simulink model "sampleModel1905_3_sub_sub_sub"  (R2023a)
settings: Solver=VariableStepAuto  StartTime=0.0  StopTime=10.0  RelTol=1e-3
libraries: hdlsllib x5
settings Model: Creator=user1  LastModifiedBy=user1

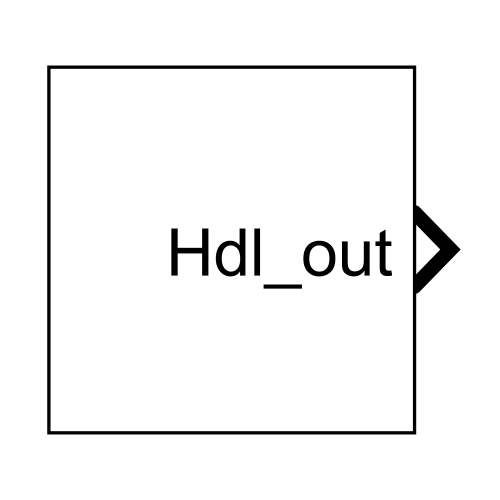
[thumbnail: Simulink's stored preview of the top-level diagram]
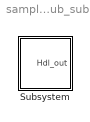
== system sampleModel1905_3_sub_sub_sub ==
  Subsystem : Subsystem

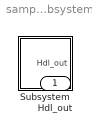
== system sampleModel1905_3_sub_sub_sub/Subsystem ==
  Subsystem : Subsystem
  Hdl_out : Outport  OutDataTypeStr=uint8

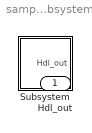
== system sampleModel1905_3_sub_sub_sub/Subsystem/Subsystem ==
  Subsystem : Subsystem
  Hdl_out : Outport  OutDataTypeStr=uint8

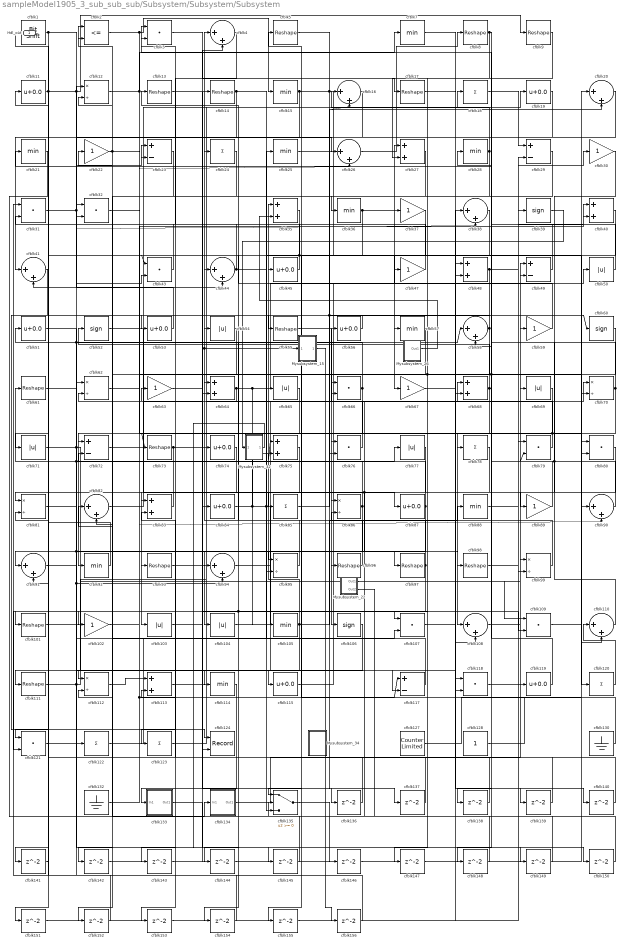
== system sampleModel1905_3_sub_sub_sub/Subsystem/Subsystem/Subsystem ==
  Mysubsystem_15 : Subsystem  TreatAsAtomicUnit=on  RTWFcnName=Mysubsystem_15
      settings: RTWFcnNameOpts=User specified  RTWFileNameOpts=Use function name
  Mysubsystem_22 : Subsystem  TreatAsAtomicUnit=on  RTWFcnName=Mysubsystem_22
      settings: RTWFcnNameOpts=User specified  RTWFileNameOpts=Use function name
  Mysubsystem_26 : Subsystem  TreatAsAtomicUnit=on  RTWFcnName=Mysubsystem_26
      settings: RTWFcnNameOpts=User specified  RTWFileNameOpts=Use function name
  Mysubsystem_32 : Subsystem  TreatAsAtomicUnit=on  RTWFcnName=Mysubsystem_32
      settings: RTWFcnNameOpts=User specified  RTWFileNameOpts=Use function name
  Mysubsystem_34 : Subsystem  TreatAsAtomicUnit=on  RTWFcnName=Mysubsystem_34
      settings: RTWFcnNameOpts=User specified  RTWFileNameOpts=Use function name
  cfblk1 : hdlsllib/Logic and Bit Operations/Bit Shift  mode=Shift Left Logical  N=0
  cfblk{5,8..9,13..14,17,55,61,73,93,96..98,101,111} (15 alike) : Reshape
  cfblk{22,30,37,47,59,63,67,89,102} (9 alike) : Gain  OutDataTypeStr=uint8
  cfblk{50,54,65,69,71,77,103..104} (8 alike) : Abs  OutDataTypeStr=uint8  SaturateOnIntegerOverflow=off
  cfblk{7,15,21,25,28,36,57,88,92,105,114} (11 alike) : MinMax  OutDataTypeStr=uint8
  cfblk{39,52,60,106} (4 alike) : Signum
  cfblk{3,31..32,43,66,76,79..80,107,109,118,121} (12 alike) : DotProduct  OutDataTypeStr=uint8
  cfblk{4,16,20,26,38,41,44,58,82,90..91,94,108,110} (14 alike) : Sum  Inputs=|++  OutDataTypeStr=uint8
  cfblk{11,19,45,51,53,56,74,84,87,115,119} (11 alike) : Bias  Bias=0.0  SaturateOnIntegerOverflow=off
  cfblk{12,62,70,81,86,95,99,112} (8 alike) : Product  Inputs=*/  OutDataTypeStr=uint8  RndMeth=Zero  SaturateOnIntegerOverflow=on
  cfblk{27,35,40,48,64,68,75,83,113} (9 alike) : Sum  OutDataTypeStr=uint8
  cfblk{23,29,49,72,117} (5 alike) : Sum  Inputs=+-  OutDataTypeStr=uint8
  cfblk{18,24,78,85,120,122..123} (7 alike) : Sum  Inputs=+  OutDataTypeStr=uint8
  cfblk124 : Record  FileSettingsInternal="{\"entries\":[{\"content\":{\"excelSettings\":{\"content\":{},\"type\":\"Streamout.ExcelSettings\"}},\"type\":\"Streamout.FileSettingStorage\",\"uuid\":\"\"}],\"packageUris\":[\"http:\\/\\/schema.mathworks.com\\/mf0\\/streamout_blocks\\/R2020a\"],\"version\":\"1.0\"}"  Layout=[1 1]  SignalsInternal="{\"entries\":[{\"content\":{\"signals\":[{\"content\":{\"blockPath\":[],\"dimensions\":[1],\"domain\":\"\",\"lineColor\":\"#a2142f\",\"plots\":[1],\"port\":1,\"signalID\":50680,\"signalName\":\"cfblk41\"},\"type\":\"RecordBlkView.Signal\",\"uuid\":\"\"},{\"content\":{\"blockPath\":[],\"dimensions\":[1],\"domain\":\"\",\"lineColor\":\"#139fff\",\"plots\":[1],\"port\":2,\"signalID\":50683,\"signalName\":\"cfblk66\"},\"type\":\"RecordBlkView.Signal\",\"uuid\":\"\"}]},\"type\":\"RecordBlkView.InputSignals\",\"uuid\":\"\"}],\"packageUris\":[\"http:\\/\\/schema.mathworks.com\\/mf0\\/streamout_blocks\\/R2020a\"],\"version\":\"1.0\"}"  VisualizationBindings="{\"xyplotplugin\":{\"info\":[{\"series\":[{\"bindingParametersList\":[{\"parameter\":\"X-Axis\",\"signalID\":50680,\"signalName\":\"cfblk41\"},{\"parameter\":\"Y-Axis\",\"signalID\":50683,\"signalName\":\"cfblk66\"}],\"seriesID\":14203}],\"subplotID\":1}]}}"  CompatibilityTag=XY  st=-1
  cfblk127 : hdlsllib/Sources/Counter Limited  uplimit=7  tsamp=-1
  cfblk128 : Constant  OutDataTypeStr=uint8  SampleTime=-1
  cfblk130 : Ground
  cfblk132 : Ground
  cfblk133 : Subsystem
      settings: LibrarySourceBlock=|
      | hdlsllib/Ports &
      | Subsystems/Subsystem
  cfblk134 : Subsystem
      settings: LibrarySourceBlock=|
      | hdlsllib/Ports &
      | Subsystems/Subsystem
  cfblk135 : Switch  OutDataTypeStr=uint8  SaturateOnIntegerOverflow=off  InputSameDT=off
  cfblk{136..156} (21 alike) : Delay  SampleTime=1
  cfblk2 : RelationalOperator  Operator=<=  OutDataTypeStr=boolean  InputSameDT=off
  Hdl_out : Outport  OutDataTypeStr=uint8
  wires:
  cfblk123/1 -> cfblk77/1
  cfblk68/1 -> cfblk152/1, cfblk28/1, cfblk52/1
  cfblk59/1 -> cfblk13/1
  cfblk96/1 -> cfblk4/1
  cfblk73/1 -> cfblk109/2, cfblk103/1
  cfblk113/1 -> cfblk19/1
  cfblk71/1 -> cfblk115/1, cfblk117/2, cfblk94/2
  cfblk102/1 -> cfblk40/1
  cfblk106/1 -> cfblk111/1
  cfblk105/1 -> cfblk114/1, cfblk88/1, cfblk35/1
  cfblk99/1 -> cfblk44/1, Mysubsystem_15/1(In1)
  cfblk2/1 -> cfblk26/2, cfblk15/1
  cfblk11/1 -> cfblk121/1, cfblk26/1, cfblk9/1
  cfblk79/1 -> cfblk73/1, cfblk5/1
  cfblk65/1 -> cfblk92/1
  cfblk26/1 -> cfblk8/1
  cfblk41/1 -> cfblk124/1
  cfblk64/1 -> cfblk62/2, cfblk105/1, cfblk50/1
  cfblk54/1 -> cfblk133/1(In1)
  cfblk115/1 -> cfblk27/1
  cfblk122/1 -> cfblk25/1
  cfblk3/1 -> cfblk17/1
  cfblk134/1(Out1) -> cfblk49/1
  cfblk21/1 -> cfblk134/1(In1)
  cfblk120/1 -> cfblk110/1
  cfblk86/1 -> cfblk155/1, cfblk65/1
  cfblk18/1 -> cfblk29/1
  cfblk57/1 -> cfblk106/1
  cfblk83/1 -> cfblk81/1
  cfblk80/1 -> cfblk86/1
  cfblk108/1 -> cfblk49/2
  cfblk93/1 -> cfblk104/1
  cfblk130/1 -> cfblk45/1
  cfblk25/1 -> cfblk120/1
  cfblk119/1 -> cfblk24/1
  cfblk30/1 -> cfblk89/1
  cfblk89/1 -> cfblk69/1
  cfblk98/1 -> cfblk39/1
  cfblk94/1 -> cfblk97/1
  cfblk109/1 -> cfblk80/1
  cfblk19/1 -> cfblk32/2
  cfblk37/1 -> cfblk55/1
  cfblk118/1 -> cfblk119/1
  cfblk52/1 -> cfblk87/1
  cfblk55/1 -> cfblk76/1
  cfblk77/1 -> cfblk135/1
  cfblk88/1 -> cfblk30/1
  cfblk14/1 -> cfblk47/1, cfblk41/1
  cfblk87/1 -> cfblk151/1, cfblk61/1
  cfblk84/1 -> cfblk75/2, cfblk68/1, cfblk118/2
  cfblk69/1 -> cfblk108/1
  cfblk82/1 -> cfblk18/1
  cfblk29/1 -> cfblk76/2
  cfblk15/1 -> cfblk135/3, cfblk16/2, cfblk67/1
  cfblk5/1 -> cfblk137/1, cfblk60/1
  cfblk70/1 -> cfblk102/1, cfblk21/1
  cfblk4/1 -> cfblk83/1
  cfblk104/1 -> cfblk70/1
  cfblk76/1 -> cfblk63/1
  cfblk12/1 -> cfblk68/2, cfblk7/1
  cfblk31/1 -> cfblk38/2, cfblk23/1
  cfblk78/1 -> cfblk95/1, cfblk96/1
  cfblk95/1 -> cfblk64/1
  cfblk97/1 -> cfblk54/1, cfblk154/1, cfblk121/2
  cfblk44/1 -> cfblk22/1, cfblk98/1
  cfblk81/1 -> cfblk95/2, cfblk122/1
  cfblk121/1 -> cfblk75/1, cfblk12/1
  cfblk53/1 -> cfblk41/2
  cfblk47/1 -> cfblk3/1
  cfblk50/1 -> cfblk3/2
  cfblk24/1 -> cfblk64/2
  cfblk111/1 -> cfblk107/2, cfblk99/1
  cfblk92/1 -> cfblk51/1
  cfblk72/1 -> cfblk14/1
  cfblk101/1 -> cfblk56/1
  cfblk48/1 -> cfblk40/2, cfblk91/1
  cfblk66/1 -> cfblk31/2, cfblk124/2
  cfblk27/1 -> cfblk36/1
  cfblk36/1 -> cfblk37/1, cfblk112/1
  cfblk45/1 -> cfblk43/1, cfblk11/1
  cfblk43/1 -> cfblk2/1
  cfblk74/1 -> cfblk123/1
  cfblk28/1 -> cfblk16/1, cfblk72/1
  cfblk128/1 -> cfblk110/2
  cfblk20/1 -> cfblk48/2
  cfblk8/1 -> cfblk148/1, cfblk147/1
  cfblk58/1 -> cfblk57/1, cfblk93/1
  cfblk32/1 -> cfblk78/1
  cfblk117/1 -> cfblk72/2
  cfblk56/1 -> cfblk53/1
  cfblk9/1 -> cfblk27/2
  cfblk112/1 -> cfblk113/1
  cfblk60/1 -> cfblk138/1, cfblk82/2, cfblk107/1
  cfblk110/1 -> cfblk79/2, cfblk59/1
  cfblk38/1 -> cfblk85/1
  cfblk67/1 -> cfblk108/2
  cfblk1/1 -> cfblk44/2, cfblk71/1
  cfblk16/1 -> cfblk101/1
  cfblk91/1 -> cfblk43/2, cfblk58/1
  cfblk90/1 -> cfblk58/2
  cfblk103/1 -> cfblk74/1
  cfblk49/1 -> cfblk23/2
  cfblk63/1 -> cfblk84/1
  cfblk7/1 -> cfblk70/2
  cfblk85/1 -> cfblk20/2
  cfblk127/1 -> cfblk90/1
  cfblk62/1 -> cfblk66/1
  cfblk22/1 -> cfblk80/2, cfblk2/2
  cfblk51/1 -> cfblk94/1
  cfblk132/1 -> cfblk117/1, cfblk90/2
  cfblk13/1 -> cfblk136/1
  cfblk136/1 -> cfblk32/1
  cfblk137/1 -> cfblk1/1
  cfblk138/1 -> cfblk112/2
  cfblk107/1 -> cfblk139/1
  cfblk139/1 -> cfblk83/2
  cfblk17/1 -> cfblk140/1
  cfblk140/1 -> cfblk113/2
  cfblk35/1 -> cfblk141/1
  cfblk141/1 -> cfblk81/2
  cfblk23/1 -> cfblk142/1
  cfblk142/1 -> cfblk4/2
  cfblk114/1 -> cfblk143/1
  cfblk143/1 -> cfblk118/1
  cfblk40/1 -> cfblk144/1
  cfblk144/1 -> cfblk48/1
  cfblk145/1 -> cfblk82/1
  cfblk135/1 -> cfblk146/1
  cfblk146/1 -> cfblk29/2
  cfblk147/1 -> cfblk20/1
  cfblk148/1 -> cfblk66/2
  cfblk133/1(Out1) -> cfblk149/1
  cfblk149/1 -> cfblk86/2
  cfblk61/1 -> cfblk150/1
  cfblk150/1 -> cfblk12/2
  cfblk151/1 -> cfblk38/1
  cfblk152/1 -> cfblk91/2
  cfblk75/1 -> cfblk153/1
  cfblk153/1 -> cfblk99/2
  cfblk154/1 -> cfblk31/1
  cfblk155/1 -> cfblk79/1
  cfblk156/1 -> cfblk62/1
  Mysubsystem_15/1(Out1) -> cfblk156/1
  Mysubsystem_22/1(Out1) -> cfblk109/1
  Mysubsystem_22/2(Out2) -> cfblk135/2
  Mysubsystem_26/1(Out1) -> cfblk35/2
  cfblk39/1 -> Mysubsystem_32/1(In1)
  Mysubsystem_32/1(Out1) -> cfblk145/1

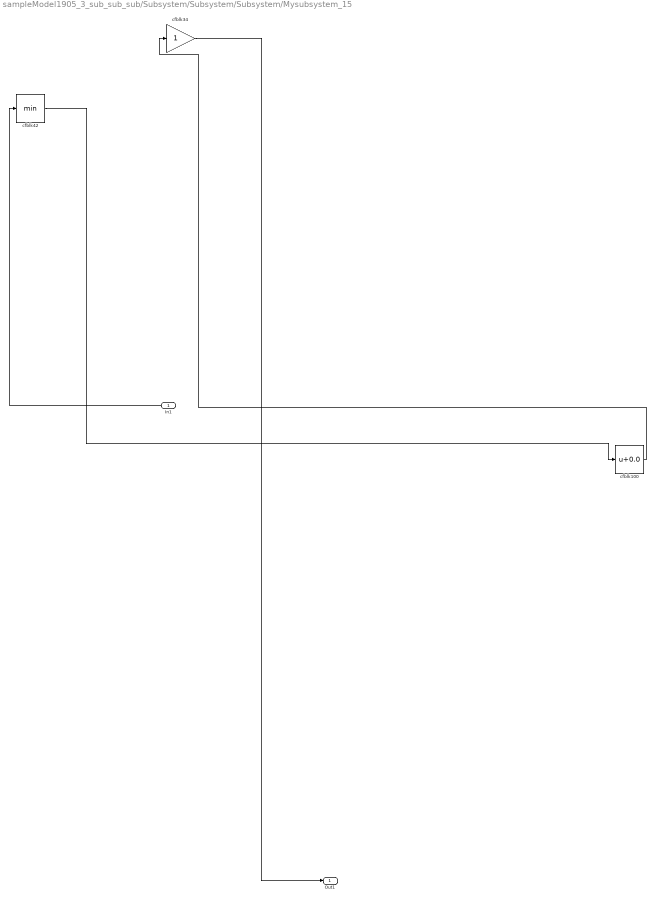
== system sampleModel1905_3_sub_sub_sub/Subsystem/Subsystem/Subsystem/Mysubsystem_15 ==
  In1 : Inport
  cfblk100 : Bias  Bias=0.0  SaturateOnIntegerOverflow=off
  cfblk34 : Gain
  cfblk42 : MinMax
  Out1 : Outport
  wires:
  cfblk34/1 -> Out1/1
  In1/1 -> cfblk42/1
  cfblk100/1 -> cfblk34/1
  cfblk42/1 -> cfblk100/1

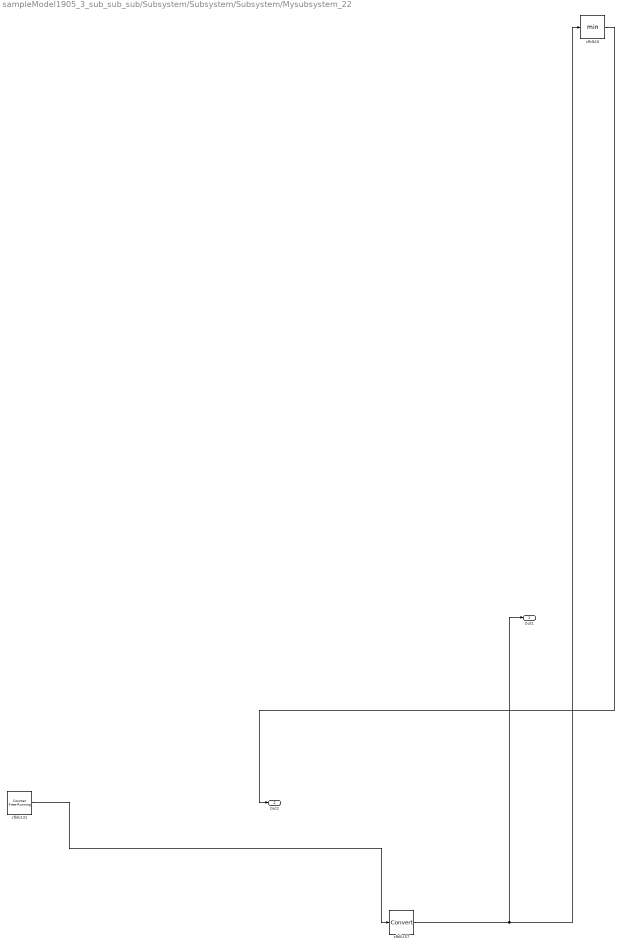
== system sampleModel1905_3_sub_sub_sub/Subsystem/Subsystem/Subsystem/Mysubsystem_22 ==
  cfblk10 : MinMax
  cfblk131 : hdlsllib/Sources/Counter Free-Running  NumBits=16  tsamp=-1
  cfblk157 : DataTypeConversion  SaturateOnIntegerOverflow=off  RndMeth=Floor
  Out1 : Outport
  Out2 : Outport  Port=2
  wires:
  cfblk131/1 -> cfblk157/1
  cfblk157/1 -> cfblk10/1, Out1/1
  cfblk10/1 -> Out2/1

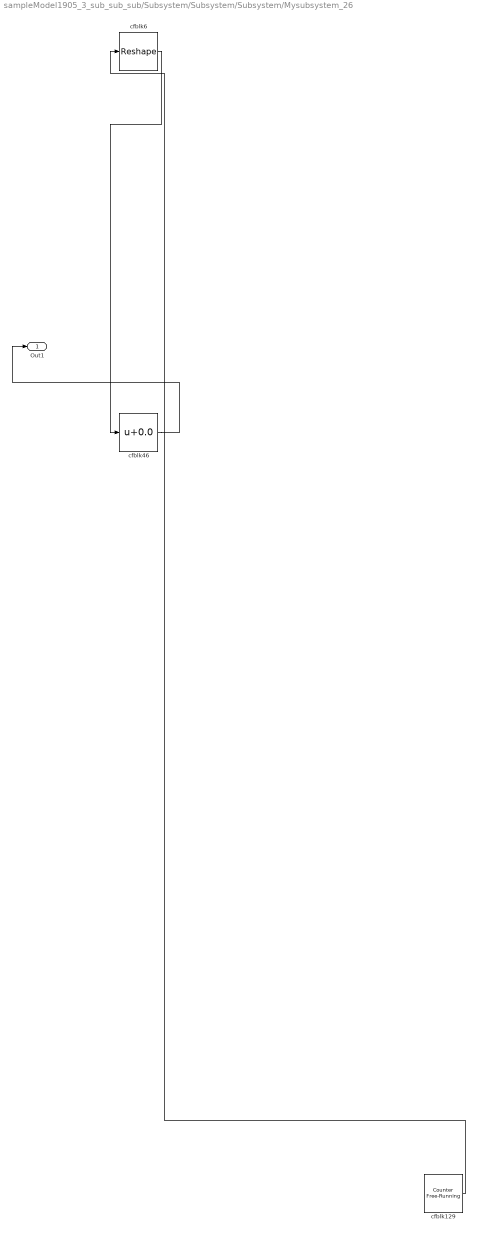
== system sampleModel1905_3_sub_sub_sub/Subsystem/Subsystem/Subsystem/Mysubsystem_26 ==
  cfblk129 : hdlsllib/Sources/Counter Free-Running  NumBits=16  tsamp=-1
  cfblk46 : Bias  Bias=0.0  SaturateOnIntegerOverflow=off
  cfblk6 : Reshape
  Out1 : Outport
  wires:
  cfblk46/1 -> Out1/1
  cfblk129/1 -> cfblk6/1
  cfblk6/1 -> cfblk46/1

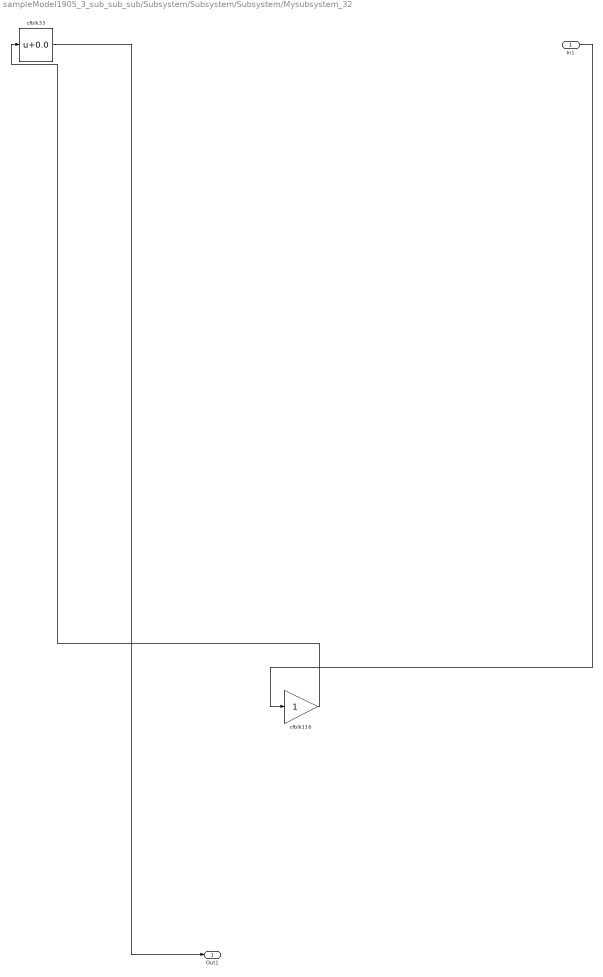
== system sampleModel1905_3_sub_sub_sub/Subsystem/Subsystem/Subsystem/Mysubsystem_32 ==
  In1 : Inport
  cfblk116 : Gain
  cfblk33 : Bias  Bias=0.0  SaturateOnIntegerOverflow=off
  Out1 : Outport
  wires:
  In1/1 -> cfblk116/1
  cfblk116/1 -> cfblk33/1
  cfblk33/1 -> Out1/1

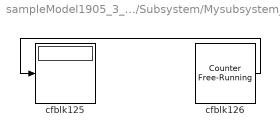
== system sampleModel1905_3_sub_sub_sub/Subsystem/Subsystem/Subsystem/Mysubsystem_34 ==
  cfblk125 : Display
  cfblk126 : hdlsllib/Sources/Counter Free-Running  NumBits=16  tsamp=-1
  wires:
  cfblk126/1 -> cfblk125/1

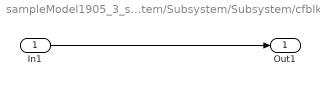
== system sampleModel1905_3_sub_sub_sub/Subsystem/Subsystem/Subsystem/cfblk133 ==
  In1 : Inport
  Out1 : Outport
  wires:
  In1/1 -> Out1/1

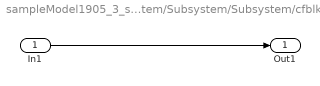
== system sampleModel1905_3_sub_sub_sub/Subsystem/Subsystem/Subsystem/cfblk134 ==
  In1 : Inport
  Out1 : Outport
  wires:
  In1/1 -> Out1/1
